simulink model "Ocean_Current_Turbine_Model_20m_v12_VarBuoy_CL_a"  (R2019a)
settings: Solver=FixedStepAuto  StartTime=0.0  StopTime=70000  FixedStep=0.0004  MaxStep=15  MinStep=0.00000000001  RelTol=1e-4
values from neighbouring files (symbols this model uses):
  rb =     [rotor_data_for_20m_fx83_varSp_varPi_P2F_GS.mat]    (also in turbine_constants_20mD_turbulence_VarBuoy.m = rotor_constants_20mD_turbulence(N_mesh); turbine_constants_20mD_turbulence_VarBuoy_v2.m = rotor_constants_20mD_turbulence(N_mesh))
undefined symbols (not defined in the file or in its folder): attachment_point, calc_cable_water_vel, controller_v2, drag_forces_20m_IBP_v3, equations_of_motion5_external_generator, equations_of_motion_cable, gravity_buoyancy_3_VarBuoy_v2, mdl
settings Model: Creator=Billy  LastModifiedBy=jvanzwi
settings DataIOCC: LimitDataPoints=on  SaveFormat=Array  SignalLoggingSaveFormat=ModelDataLogs
settings OptimizationCC: ExpressionDepthLimit=2147483647  LifeSpan=inf
settings DebuggingCC: UnderspecifiedInitializationDetection=Classic  MergeDetectMultiDrivingBlocksExec=none  SolverPrmCheckMsg=warning  InheritedTsInSrcMsg=none  MultiTaskDSMMsg=warning  MultiTaskCondExecSysMsg=none  FcnCallInpInsideContextMsg=warning  AllowSymbolicDim=off  StateNameClashWarn=warning  SFUnexpectedBacktrackingDiag=warning  SFNoUnconditionalDefaultTransitionDiag=warning  SFExecutionAtInitializationDiag=none  ArithmeticOperatorsInVariantConditions=warning
settings HardwareCC: ProdBitPerPointer=32  ProdBitPerSizeT=32  ProdBitPerPtrDiffT=32  ProdLargestAtomicFloat=None  ProdIntDivRoundTo=Undefined  ProdEndianess=Unspecified  ProdWordSize=32  ProdHWDeviceType=32-bit Generic
settings ModelReferenceCC: PropagateSignalLabelsOutOfModel=off
settings SFSimCC: SimUseLocalCustomCode=off
settings RTWCC: RTWUseLocalCustomCode=off
settings CodeAppCC: StateflowObjectComments=on
settings GRTTargetCC: TargetLangStandard=C89/C90 (ANSI)  GeneratePreprocessorConditionals=Disable all  CombineOutputUpdateFcns=off  GRTInterface=on
settings ConfigComp: CovMetricSettings=dw  CovHtmlReporting=on  CovSaveCumulativeToWorkspaceVar=on  CovSaveSingleToWorkspaceVar=on  CovExternalEMLEnable=off  CovSFcnEnable=off

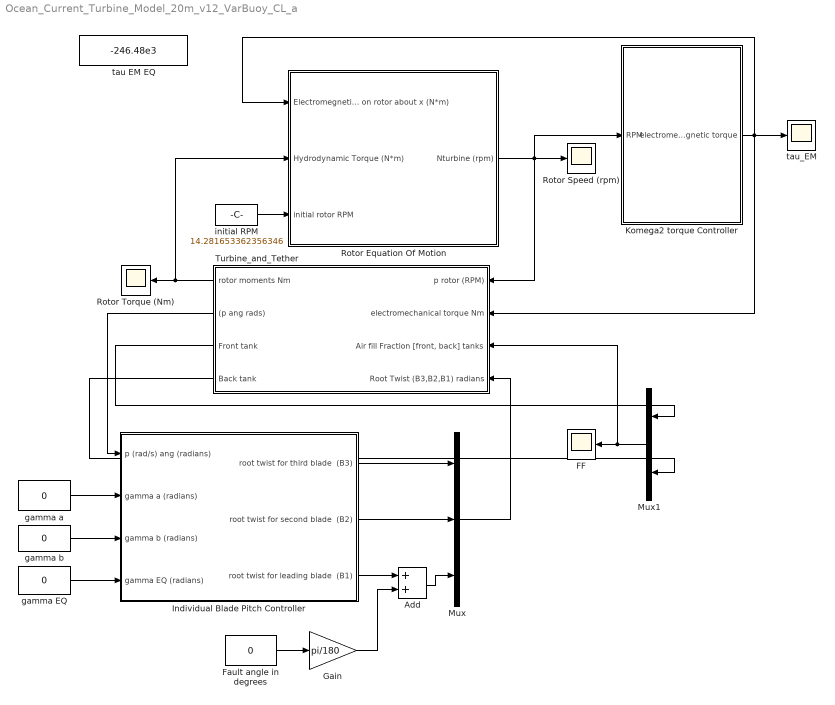
== system Ocean_Current_Turbine_Model_20m_v12_VarBuoy_CL_a ==
  Add : Sum
  FF : Scope
  Fault angle in degrees : Constant  Value=0
  Gain : Gain  Gain=pi/180
  Individual Blade Pitch Controller : Subsystem
  Komega2 torque Controller : Subsystem  mask{C_pmax=0.55, TSR_max=10.14}
      mask prompts: C_pmax "Enter maximum Cp for rotor"; TSR_max "Enter TSR associated with Cp max"
  Mux : Mux  Inputs=3
  Mux1 : Mux  Inputs=2
  Rotor Equation Of Motion : Subsystem
      mask init:
      | N_mesh = 32;
      | %this loads all of the constants that define the turbine
      | [mdl rb] = turbine_constants_20mD_turbulence_VarBuoy(N_mesh);
  Rotor Speed (rpm) : Scope
  Rotor Torque (Nm) : Scope
  Turbine_and_Tether : Subsystem  mask{L_cable=91*20/3, D_cable=0.16, m_cable=46, disp_m_cable=20.6, EA_cable=8800000*400/9, Cd_cable=1.5, N_mesh=16, U=1.6, dUdZ=-1.6/325, N_cable=5, Hs=5, TI=0.37, Z_disp=0, Y_disp=0, inflowSelection=1}
      mask prompts: L_cable "total length of cable attached to nose cone [m] (91)"; D_cable "Diamiter of the cable attached to the nose cone [m] (0.0127)"; m_cable "mass of cable per meter lenght [kg] (0.7143)"; disp_m_cable "displaced mass of cable per meter lenght [kg] (0.11)"; EA_cable "Stiffness of cable (EA) [m/N] (2.2e6)"; Cd_cable "drag coeficient for the cable [1.5]"; N_mesh "Number of mesh points in the grid (10-40)"; U "water speed (m/s)"; dUdZ "water speed gradient dUdZ (0 or -U/325)"; N_cable "Number of cable elements"; Hs "Significant wave height (m)"; TI "Turbulence Intensity as a fraction"; Z_disp "Turbine displacement from equilibrium in Z (down) [m]"; Y_disp "Turbine displacement from equilibrium in Y [m]"; inflowSelection "Flag to turn on (1) or off (0) the ADCP section"
      mask init:
      | [mdl rb] = turbine_constants_20mD_turbulence_VarBuoy_v2(N_mesh);
      | Z0_ZCAP = 325;
      | %initial try for v11
      | %this is for 1.6 m/s
      | state0 = [0, 0, 0, 0, 0, 0, 555.8476,1.6924+Y_disp, 75+Z_disp, 0.0073, 0.0189, 3.1485]; %v1
      | %state0 = [0, 0, 0, 0, 0, 0, 489.61, -139.45, 50, 0.010026, 0.059407, 3.084005]; %v2
      | %state0 = [0, 0, 0, 0, 0, 0, 497, -120, 50, 0.0085, 0.064, 3.048]; %v3
      | %state0 = [0, 0, 0, 0, 0, 0, 473, -93, 50, 0.0027, 0.0687, 3.339]; %v4 
      | 
      | Current=[U; 0; 0; dUdZ; 0; 0];%Current speed vector
      | 
      | first_node = [0 0 0 0 0 Z0_ZCAP];
      | last_node = attachment_point([state0(1:4),0,state0(5:10),0,state0(11:12)],mdl);
      | if N_cable == 1;
      |     state_cable0 = []; %intermediate nodes
      | elseif N_cable == 2;
      |     state_cable0 = 0.5*last_node+0.5*first_node;
      | elseif N_cable == 3;
      |     state_cable0 = [0.3333*last_node+0.6666*first_node 0.6666*last_node+0.3333*first_node];
      | elseif N_cable == 4;
      |     state_cable0 = [0.25*last_node+0.75*first_node 0.5*last_node+0.5*first_node 0.75*last_node+0.25*first_node];
      | elseif N_cable == 5;
      |     state_cable0 = [0.2*last_node+0.8*first_node 0.4*last_node+0.6*first_node 0.6*last_node+0.4*first_node 0.8*last_node+0.2*first_node];
      | elseif N_cable == 8;
      |     state_cable0 = [0.125*last_node+0.8750*first_node 0.25*last_node+0.75*first_node 0.375*last_node+0.625*first_node 0.5*last_node+0.5*first_node 0.625*last_node+0.375*first_node 0.75*last_node+0.25*first_node 0.878*last_node+0.125*first_node];
      | else
      |     disp('cable model curently only valid for 1-5 elements')
      | end
      |     
      | Mod_vars.l = L_cable;
      | Mod_vars.D = D_cable;
      | Mod_vars.m = m_cable;
      | Mod_vars.disp_m = disp_m_cable;
      | Mod_vars.N_cable = N_cable;
      | Mod_vars.EA = EA_cable;
      | Mod_vars.Cd = Cd_cable;
      | Mod_vars.drag_t = 1/4*mdl.rho*2*pi*Mod_vars.D/2*Mod_vars.l*Mod_vars.Cd;
      | Mod_vars.drag_n = 1/4*mdl.rho*Mod_vars.D*Mod_vars.l*Mod_vars.Cd;
      | Mod_vars.K = Mod_vars.EA/Mod_vars.l;
      | Mod_vars.Wt = (Mod_vars.m*mdl.g-Mod_vars.disp_m*mdl.g)*Mod_vars.l;
      | Mod_vars.M = Mod_vars.m*Mod_vars.l;
      | Mod_vars.Cid = 1000;
      | Mod_vars.rho = mdl.rho;
      | Mod_vars.Z0_ZCAP = Z0_ZCAP;
      | Mod_vars.Current=Current;
      | 
      | %% This calls the wave spectrum that is used
      | n=50; %number of wave elements
      | m=7;  %number of wave directions
      | %Hs=0;%1.859; %significant wave height
      | angle0=180+90; %mean direction of wave propagation
      | s=25; %not sure
      | waves = waves_spec_calc2(n,m,Hs,angle0,s);
      | 
      | %% This is what calculates all of the turbulence constants
      | %TI = 0.10; %Turbulence intensity
      | a=1;b=1; %sigma_y=a*sigma_x,sigma_z=b*sigma_x
      | fmin = 1/60/60;%minimum frequency to resolve
      | fmax=10; %maximum frequency to resolve
      | C=27; %coherence decay constant, Veers (1986)
      | % N=round(2*fmax*T*1.2); %data points
      | P=1500;%number of frequency discretization
      | turbulence = turbulence_constants_v3(TI,fmin,fmax,rb.radius,N_mesh,U,a,b,C,P); %this creates the required wave data
      | 
      | %% This section processes ADCP data and outputs current velocities
      | filename = 'ADCP-Data-Irma.mat'; %Input file with ADCP data
      | %tStart = datenum('25-Sep-0017 18:00:00');%start time for generating a subset of data v1
      | tStart = datenum('11-Sep-0017 10:00:00');%start time for generating a subset of data v2
      | %tStart = datenum('26-Sep-0017 00:32:00');%start time for generating a subset of data v3
      | %tStart = datenum('26-Sep-0017 00:55:00');%start time for generating a subset of data v4
      | tStop = datenum('13-Sep-0017 10:00:00');%stop time for generating a subset of data
      | %tmin - 06-Sep-0017 21:08:00
      | %tmax - 04-Nov-0017 18:14:00
      | ADCP = ADCP_Init(filename,tStart,tStop,inflowSelection)
  gamma EQ : Constant  Value=0
  gamma a : Constant  Value=0
  gamma b : Constant  Value=0
  initial RPM : Constant  Value=14.281653362356346
  tau EM EQ : Constant  Value=-246.48e3
  tau_EM : Scope
  wires:
  Rotor Equation Of Motion/1(Nturbine (rpm)) -> Rotor Speed (rpm)/1, Komega2 torque Controller/1(RPM), Turbine_and_Tether/1(p rotor (RPM))
  Mux/1 -> Turbine_and_Tether/4(Root Twist (B3,B2,B1) radians)
  Turbine_and_Tether/1(rotor moments Nm) -> Rotor Equation Of Motion/2(Hydrodynamic Torque (N*m)), Rotor Torque (Nm)/1
  Turbine_and_Tether/2((p ang rads)) -> Individual Blade Pitch Controller/1(p (rad/s) ang (radians))
  Individual Blade Pitch Controller/1(root twist for third blade  (B3)) -> Mux/1
  Individual Blade Pitch Controller/2(root twist for second blade  (B2)) -> Mux/2
  gamma EQ/1 -> Individual Blade Pitch Controller/4(gamma EQ (radians))
  initial RPM/1 -> Rotor Equation Of Motion/3(initial rotor RPM)
  gamma a/1 -> Individual Blade Pitch Controller/2(gamma a (radians))
  gamma b/1 -> Individual Blade Pitch Controller/3("gamma b (radians) ")
  Komega2 torque Controller/1(electromegnetic torque) -> Turbine_and_Tether/2(electromechanical torque Nm), tau_EM/1, Rotor Equation Of Motion/1(Electromegnetic Torque  on rotor about x (N*m))
  Mux1/1 -> Turbine_and_Tether/3("Air fill Fraction [front, back] tanks"), FF/1
  Fault angle in degrees/1 -> Gain/1
  Individual Blade Pitch Controller/3(root twist for leading blade  (B1)) -> Add/1
  Add/1 -> Mux/3
  Gain/1 -> Add/2
  Turbine_and_Tether/3(Front tank) -> Mux1/1
  Turbine_and_Tether/4(Back tank) -> Mux1/2

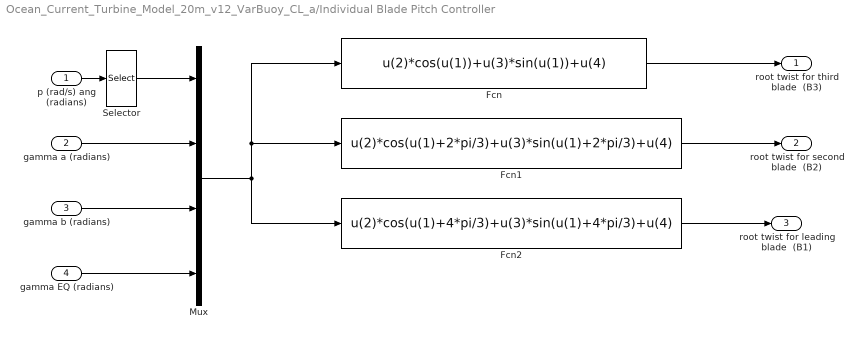
== system Ocean_Current_Turbine_Model_20m_v12_VarBuoy_CL_a/Individual Blade Pitch Controller ==
  p (rad/s) ang (radians) : Inport
  gamma a (radians) : Inport  Port=2
  "gamma b (radians) " : Inport  Port=3
  gamma EQ (radians) : Inport  Port=4
  Fcn : Fcn  Expr=u(2)*cos(u(1))+u(3)*sin(u(1))+u(4)
  Fcn1 : Fcn  Expr=u(2)*cos(u(1)+2*pi/3)+u(3)*sin(u(1)+2*pi/3)+u(4)
  Fcn2 : Fcn  Expr=u(2)*cos(u(1)+4*pi/3)+u(3)*sin(u(1)+4*pi/3)+u(4)
  Mux : Mux
  Selector : Selector  InputPortWidth=2  IndexOptions=Index vector (dialog)  Indices=2  OutputSizes=1
  root twist for third blade  (B3) : Outport
  root twist for second blade  (B2) : Outport  Port=2
  root twist for leading blade  (B1) : Outport  Port=3
  wires:
  Fcn/1 -> root twist for third blade  (B3)/1
  Fcn1/1 -> root twist for second blade  (B2)/1
  Fcn2/1 -> root twist for leading blade  (B1)/1
  p (rad/s) ang (radians)/1 -> Selector/1
  Selector/1 -> Mux/1
  gamma a (radians)/1 -> Mux/2
  "gamma b (radians) "/1 -> Mux/3
  Mux/1 -> Fcn/1, Fcn1/1, Fcn2/1
  gamma EQ (radians)/1 -> Mux/4

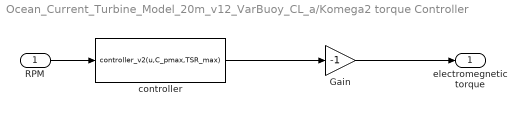
== system Ocean_Current_Turbine_Model_20m_v12_VarBuoy_CL_a/Komega2 torque Controller ==
  RPM : Inport
  Gain : Gain  Gain=-1
  controller : MATLABFcn  Description=This block calls the rotor code that calculates the hydrodynamic forces on the rotor  MATLABFcn=controller_v2(u,C_pmax,TSR_max)  OutputDimensions=1  SampleTime=0.05
  electromegnetic torque : Outport
  wires:
  RPM/1 -> controller/1
  controller/1 -> Gain/1
  Gain/1 -> electromegnetic torque/1

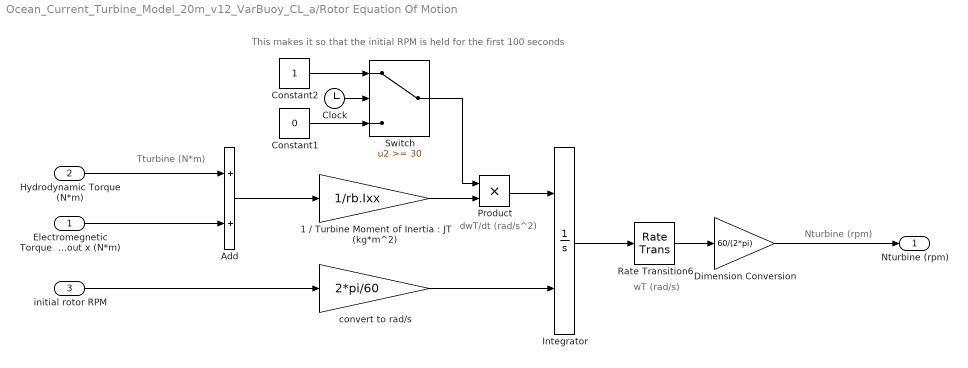
== system Ocean_Current_Turbine_Model_20m_v12_VarBuoy_CL_a/Rotor Equation Of Motion ==
  note: This makes it so that the initial RPM is held for the first 100 seconds
  note: Tturbine (N*m)
  note: dwT/dt (rad/s^2)
  note: wT (rad/s)
  note: Nturbine (rpm)
  Electromegnetic Torque  on rotor about x (N*m) : Inport
  Hydrodynamic Torque (N*m) : Inport  Port=2
  initial rotor RPM : Inport  Port=3
  "1 / Turbine Moment of Inertia : JT (kg*m^2)" : Gain  Gain=1/rb.Ixx
  Add : Sum
  Clock : Clock
  Constant1 : Constant  Value=0
  Constant2 : Constant
  Dimension Conversion : Gain  Gain=60/(2*pi)
  Integrator : Integrator  InitialConditionSource=external
  Product : Product
  Rate Transition6 : RateTransition  OutPortSampleTime=0.05
  Switch : Switch  Threshold=30
  convert to rad/s : Gain  Gain=2*pi/60
  Nturbine (rpm) : Outport
  wires:
  Hydrodynamic Torque (N*m)/1 -> Add/1
  Integrator/1 -> Rate Transition6/1
  Dimension Conversion/1 -> Nturbine (rpm)/1
  convert to rad/s/1 -> Integrator/2
  Add/1 -> "1 / Turbine Moment of Inertia : JT (kg*m^2)"/1
  Electromegnetic Torque  on rotor about x (N*m)/1 -> Add/2
  Rate Transition6/1 -> Dimension Conversion/1
  initial rotor RPM/1 -> convert to rad/s/1
  Clock/1 -> Switch/2
  Constant1/1 -> Switch/3
  Constant2/1 -> Switch/1
  Product/1 -> Integrator/1
  "1 / Turbine Moment of Inertia : JT (kg*m^2)"/1 -> Product/2
  Switch/1 -> Product/1

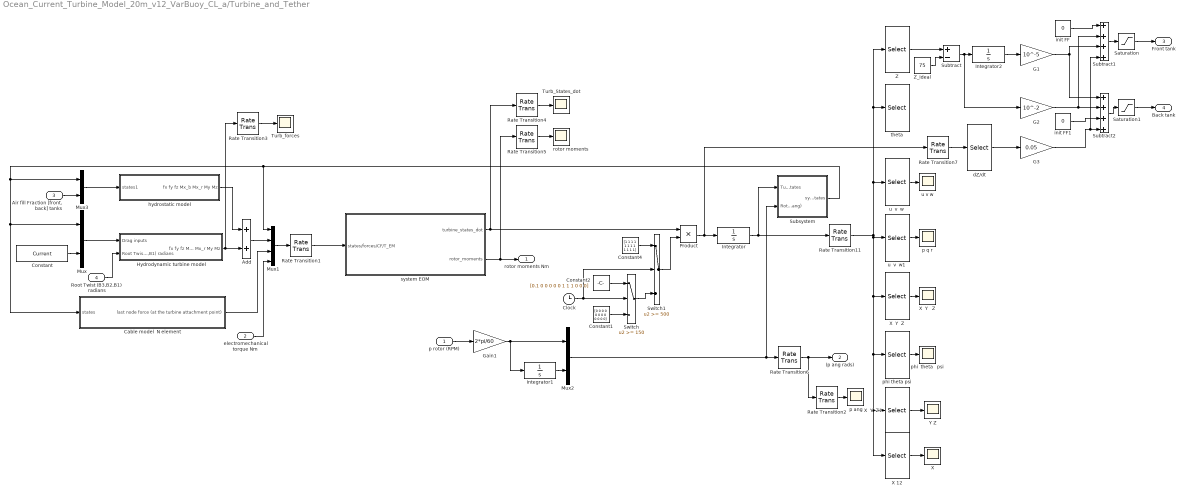
== system Ocean_Current_Turbine_Model_20m_v12_VarBuoy_CL_a/Turbine_and_Tether ==
  p rotor (RPM) : Inport
  electromechanical torque Nm : Inport  Port=2
  "Air fill Fraction [front, back] tanks" : Inport  Port=3
  Root Twist (B3,B2,B1) radians : Inport  Port=4
  " Z" : Selector  InputPortWidth=12  IndexOptions=Index vector (dialog)  Indices=9  OutputSizes=1
  " dZ/dt" : Selector  InputPortWidth=12  IndexOptions=Index vector (dialog)  Indices=9  OutputSizes=1
  Add : Sum
  Cable model  N element : Subsystem
  Clock : Clock
  Constant : Constant  Value=Current
  Constant1 : Constant  Value=[0 0 0 0 0 0 0 0 0 0 0 0]
  Constant2 : Constant  Value=[0.1 0 0 0 0 0 1 1 1 0 0 0]
  Constant4 : Constant  Value=[1 1 1 1 1 1 1 1 1 1 1 1]
  G1 : Gain  Gain=10^-5
  G2 : Gain  Gain=10^-2
  G3 : Gain  Gain=0.05
  Gain1 : Gain  Gain=2*pi/60
  Hydrodynamic turbine model : Subsystem
  Integrator : Integrator  InitialCondition=state0  ContinuousStateAttributes='states'
  Integrator1 : Integrator  ContinuousStateAttributes='states'
  Integrator2 : Integrator  ContinuousStateAttributes='intZ'
  Mux : Mux  Inputs=2
  Mux1 : Mux
  Mux2 : Mux  Inputs=2
  Mux3 : Mux  Inputs=2
  Product : Product
  Rate Transition1 : RateTransition  OutPortSampleTime=0.05
  Rate Transition{2..5,7,11} (6 alike) : RateTransition  OutPortSampleTime=0.1
  Rate Transition6 : RateTransition  OutPortSampleTime=0.05
  Saturation : Saturate  UpperLimit=1
  Saturation1 : Saturate  UpperLimit=1
  Subsystem : Subsystem
  Subtract : Sum  Inputs=+-
  Subtract1 : Sum  Inputs=++++
  Subtract2 : Sum  Inputs=++++
  Switch : Switch  Threshold=150
  Switch1 : Switch  Threshold=500
  Turb_States_dot : Scope
  Turb_forces : Scope
  X : Scope
  X  Y   Z : Scope
  X  Y  Z : Selector  InputPortWidth=12  IndexOptions=Index vector (dialog)  Indices=7:9  OutputSizes=1
  X  Y  Z1 : Selector  InputPortWidth=12  IndexOptions=Index vector (dialog)  Indices=8:9  OutputSizes=1
  X 12 : Selector  InputPortWidth=12  IndexOptions=Index vector (dialog)  Indices=7  OutputSizes=1
  Y Z : Scope
  Z_ideal : Constant  Value=75
  hydrostatic model : Subsystem
  init FF : Constant  Value=0
  init FF1 : Constant  Value=0
  p ang : Scope
  p q r : Scope
  phi  theta   psi : Scope
  phi theta psi : Selector  InputPortWidth=12  IndexOptions=Index vector (dialog)  Indices=10:12  OutputSizes=1
  rotor moments : Scope
  system EOM : Subsystem
  theta : Selector  InputPortWidth=12  IndexOptions=Index vector (dialog)  Indices=11  OutputSizes=1
  u  v  w : Selector  InputPortWidth=12  IndexOptions=Index vector (dialog)  Indices=1:3  OutputSizes=1
  u  v  w1 : Selector  InputPortWidth=12  IndexOptions=Index vector (dialog)  Indices=4:6  OutputSizes=1
  u v w : Scope
  rotor moments Nm : Outport
  (p ang rads) : Outport  Port=2
  Front tank : Outport  Port=3
  Back tank : Outport  Port=4
  wires:
  phi theta psi/1 -> phi  theta   psi/1
  X  Y  Z/1 -> X  Y   Z/1
  u  v  w/1 -> u v w/1
  Hydrodynamic turbine model/1(fx fy fz Mx_b Mx_r My Mz) -> Add/2, Rate Transition3/1
  hydrostatic model/1(fx fy fz Mx_b Mx_r My Mz) -> Add/1
  Add/1 -> Mux1/2
  Mux/1 -> Hydrodynamic turbine model/1(Drag inputs)
  Constant/1 -> Mux/2
  Subsystem/1(system states) -> Mux1/1, Mux/1, Cable model  N element/1(states), Mux3/1
  Cable model  N element/1(last node force (at the turbine attachment point)) -> Mux1/3
  p rotor (RPM)/1 -> Gain1/1
  Integrator1/1 -> Mux2/2
  electromechanical torque Nm/1 -> Mux1/4
  Integrator/1 -> Rate Transition11/1, Subsystem/1(Turb States)
  Mux1/1 -> Rate Transition1/1
  system EOM/2(rotor_moments) -> rotor moments Nm/1, Rate Transition5/1
  system EOM/1(turbine_states_dot) -> Rate Transition4/1, Product/1
  Mux2/1 -> Subsystem/2(Rotor States (p ang)), Rate Transition6/1
  Gain1/1 -> Mux2/1, Integrator1/1
  Rate Transition1/1 -> system EOM/1(states/forces/CF/T_EM)
  Root Twist (B3,B2,B1) radians/1 -> Hydrodynamic turbine model/2(Root Twist (B3,B2,B1) radians)
  Rate Transition2/1 -> p ang/1
  Rate Transition3/1 -> Turb_forces/1
  Rate Transition4/1 -> Turb_States_dot/1
  Rate Transition5/1 -> rotor moments/1
  Rate Transition6/1 -> Rate Transition2/1, (p ang rads)/1
  Product/1 -> Rate Transition7/1, Integrator/1
  Constant1/1 -> Switch/3
  Constant2/1 -> Switch/1
  X  Y  Z1/1 -> Y Z/1
  u  v  w1/1 -> p q r/1
  Clock/1 -> Switch/2, Switch1/2
  Switch/1 -> Switch1/3
  Constant4/1 -> Switch1/1
  Switch1/1 -> Product/2
  Mux3/1 -> hydrostatic model/1(states1)
  "Air fill Fraction [front, back] tanks"/1 -> Mux3/2
  X 12/1 -> X/1
  Subtract2/1 -> Saturation1/1
  Subtract1/1 -> Saturation/1
  Subtract/1 -> G2/1, Integrator2/1
  " Z"/1 -> Subtract/1
  Z_ideal/1 -> Subtract/2
  Rate Transition11/1 -> X 12/1, X  Y  Z1/1, phi theta psi/1, X  Y  Z/1, u  v  w1/1, " Z"/1, theta/1, u  v  w/1
  Integrator2/1 -> G1/1
  init FF/1 -> Subtract1/1
  init FF1/1 -> Subtract2/3
  Saturation/1 -> Front tank/1
  Saturation1/1 -> Back tank/1
  G1/1 -> Subtract2/1, Subtract1/3
  G2/1 -> Subtract1/2, Subtract2/2
  Rate Transition7/1 -> " dZ/dt"/1
  " dZ/dt"/1 -> G3/1
  G3/1 -> Subtract1/4, Subtract2/4

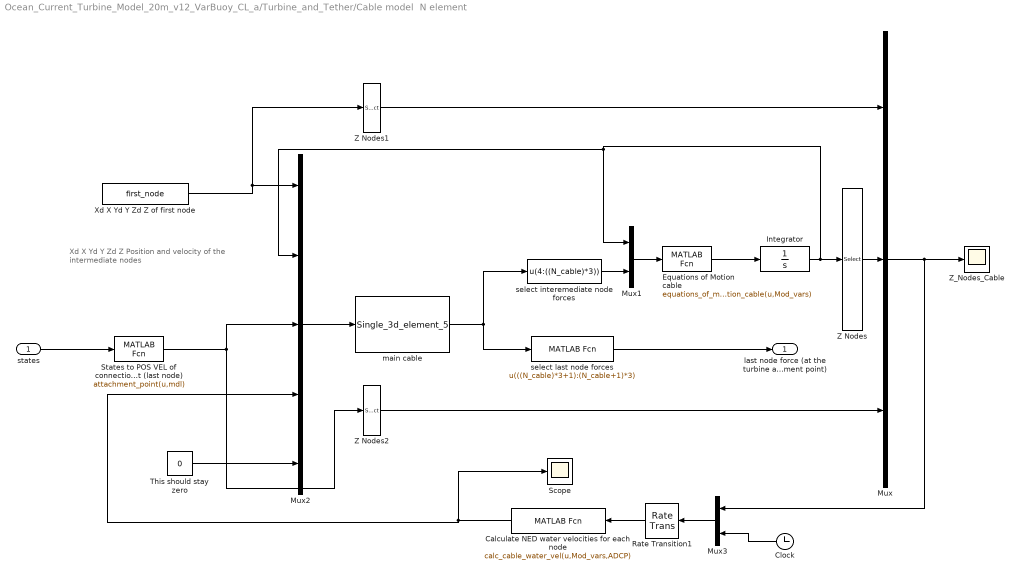
== system Ocean_Current_Turbine_Model_20m_v12_VarBuoy_CL_a/Turbine_and_Tether/Cable model  N element ==
  note: Xd X Yd Y Zd Z
      | Position and velocity of the intermediate nodes
  states : Inport
  Calculate NED water velocities for each node : MATLABFcn  MATLABFcn=calc_cable_water_vel(u,Mod_vars,ADCP)  OutputDimensions=3*(Mod_vars.N_cable+1)
  Clock : Clock
  Equations of Motion cable : MATLABFcn  MATLABFcn=equations_of_motion_cable(u,Mod_vars)  OutputDimensions=24
  Integrator : Integrator  InitialCondition=state_cable0  ContinuousStateAttributes='states_cable'
  Mux : Mux  Inputs=3
  Mux1 : Mux  Inputs=2
  Mux2 : Mux  Inputs=5
  Mux3 : Mux  Inputs=2
  Rate Transition1 : RateTransition  InitialCondition=100  OutPortSampleTime=0.1
  Scope : Scope
  States to POS VEL of connection point (last node) : MATLABFcn  MATLABFcn=attachment_point(u,mdl)
  This should stay zero : Constant  Value=0
  Xd X Yd Y Zd Z of first node : Constant  Value=first_node
  Z Nodes : Selector  InputPortWidth=24  IndexOptions=Index vector (dialog)  Indices=[6,12,18,24]  OutputSizes=1
  Z Nodes1 : Selector  InputPortWidth=6  IndexOptions=Index vector (dialog)  Indices=6  OutputSizes=1
  Z Nodes2 : Selector  InputPortWidth=6  IndexOptions=Index vector (dialog)  Indices=6  OutputSizes=1
  Z_Nodes_Cable : Scope
  main cable : S-Function  FunctionName=Single_3d_element_5  Parameters=Mod_vars  SFunctionDeploymentMode=off  EnableBusSupport=off
  select interemediate node forces : MATLABFcn  MATLABFcn=u(4:((N_cable)*3))
  select last node forces : MATLABFcn  MATLABFcn=u(((N_cable)*3+1):(N_cable+1)*3)
  last node force (at the turbine attachment point) : Outport
  wires:
  Mux1/1 -> Equations of Motion cable/1
  select interemediate node forces/1 -> Mux1/2
  States to POS VEL of connection point (last node)/1 -> Z Nodes2/1, Mux2/3
  states/1 -> States to POS VEL of connection point (last node)/1
  Xd X Yd Y Zd Z of first node/1 -> Z Nodes1/1, Mux2/1
  select last node forces/1 -> last node force (at the turbine attachment point)/1
  Equations of Motion cable/1 -> Integrator/1
  This should stay zero/1 -> Mux2/5
  Integrator/1 -> Mux2/2, Mux1/1, Z Nodes/1
  Z Nodes/1 -> Mux/2
  Z Nodes1/1 -> Mux/1
  Mux/1 -> Mux3/1, Z_Nodes_Cable/1
  Z Nodes2/1 -> Mux/3
  Mux2/1 -> main cable/1
  main cable/1 -> select interemediate node forces/1, select last node forces/1
  Calculate NED water velocities for each node/1 -> Mux2/4, Scope/1
  Mux3/1 -> Rate Transition1/1
  Clock/1 -> Mux3/2
  Rate Transition1/1 -> Calculate NED water velocities for each node/1

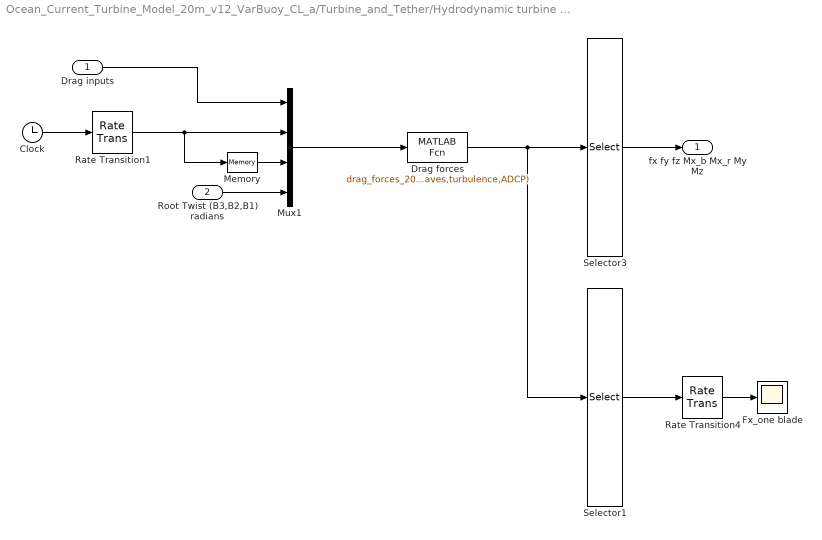
== system Ocean_Current_Turbine_Model_20m_v12_VarBuoy_CL_a/Turbine_and_Tether/Hydrodynamic turbine model ==
  Drag inputs : Inport
  Root Twist (B3,B2,B1) radians : Inport  Port=2
  Clock : Clock
  Drag forces : MATLABFcn  MATLABFcn=drag_forces_20m_IBP_v3(u,mdl,rb,waves,turbulence,ADCP)  SampleTime=0.05
  Fx_one blade : Scope
  Memory : Memory  InitialCondition=-0.05  InheritSampleTime=on
  Mux1 : Mux
  Rate Transition1 : RateTransition  OutPortSampleTime=0.05
  Rate Transition4 : RateTransition  OutPortSampleTime=0.1
  Selector1 : Selector  InputPortWidth=14  IndexOptions=Index vector (dialog)  Indices=14  OutputSizes=1
  Selector3 : Selector  InputPortWidth=14  IndexOptions=Index vector (dialog)  Indices=1:7  OutputSizes=1
  fx fy fz Mx_b Mx_r My Mz : Outport
  wires:
  Memory/1 -> Mux1/3
  Drag inputs/1 -> Mux1/1
  Selector3/1 -> fx fy fz Mx_b Mx_r My Mz/1
  Root Twist (B3,B2,B1) radians/1 -> Mux1/4
  Mux1/1 -> Drag forces/1
  Drag forces/1 -> Selector1/1, Selector3/1
  Clock/1 -> Rate Transition1/1
  Rate Transition1/1 -> Memory/1, Mux1/2
  Rate Transition4/1 -> Fx_one blade/1
  Selector1/1 -> Rate Transition4/1

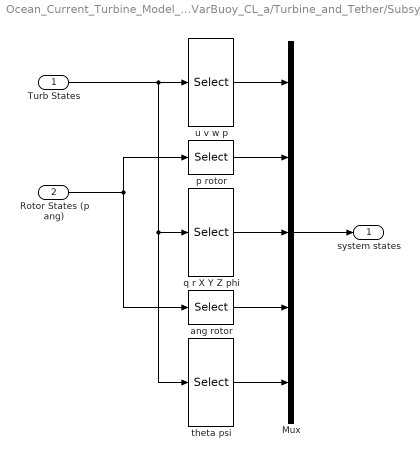
== system Ocean_Current_Turbine_Model_20m_v12_VarBuoy_CL_a/Turbine_and_Tether/Subsystem ==
  Turb States : Inport
  Rotor States (p ang) : Inport  Port=2  PortDimensions=2
  Mux : Mux  Inputs=5
  ang rotor : Selector  InputPortWidth=2  IndexOptions=Index vector (dialog)  Indices=2  OutputSizes=1
  p rotor : Selector  InputPortWidth=2  IndexOptions=Index vector (dialog)  Indices=1  OutputSizes=1
  q r X Y Z phi : Selector  InputPortWidth=12  IndexOptions=Index vector (dialog)  Indices=5:10  OutputSizes=1
  theta psi : Selector  InputPortWidth=12  IndexOptions=Index vector (dialog)  Indices=11:12  OutputSizes=1
  u v w p : Selector  InputPortWidth=12  IndexOptions=Index vector (dialog)  Indices=1:4  OutputSizes=1
  system states : Outport
  wires:
  Mux/1 -> system states/1
  theta psi/1 -> Mux/5
  ang rotor/1 -> Mux/4
  q r X Y Z phi/1 -> Mux/3
  p rotor/1 -> Mux/2
  u v w p/1 -> Mux/1
  Rotor States (p ang)/1 -> ang rotor/1, p rotor/1
  Turb States/1 -> theta psi/1, q r X Y Z phi/1, u v w p/1

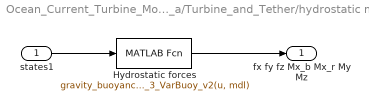
== system Ocean_Current_Turbine_Model_20m_v12_VarBuoy_CL_a/Turbine_and_Tether/hydrostatic model ==
  states1 : Inport
  Hydrostatic forces : MATLABFcn  MATLABFcn=gravity_buoyancy_3_VarBuoy_v2(u, mdl)  SampleTime=0.05
  fx fy fz Mx_b Mx_r My Mz : Outport
  wires:
  states1/1 -> Hydrostatic forces/1
  Hydrostatic forces/1 -> fx fy fz Mx_b Mx_r My Mz/1

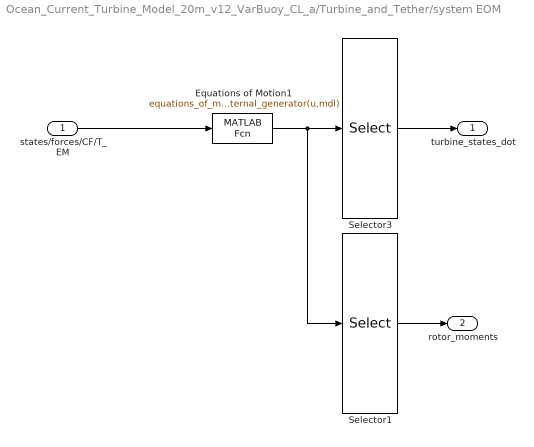
== system Ocean_Current_Turbine_Model_20m_v12_VarBuoy_CL_a/Turbine_and_Tether/system EOM ==
  states/forces/CF/T_EM : Inport
  Equations of Motion1 : MATLABFcn  MATLABFcn=equations_of_motion5_external_generator(u,mdl)  OutputDimensions=13  SampleTime=0.05
  Selector1 : Selector  InputPortWidth=13  IndexOptions=Index vector (dialog)  Indices=13  OutputSizes=1
  Selector3 : Selector  InputPortWidth=13  IndexOptions=Index vector (dialog)  Indices=1:12  OutputSizes=1
  turbine_states_dot : Outport
  rotor_moments : Outport  Port=2
  wires:
  Selector1/1 -> rotor_moments/1
  Selector3/1 -> turbine_states_dot/1
  Equations of Motion1/1 -> Selector1/1, Selector3/1
  states/forces/CF/T_EM/1 -> Equations of Motion1/1
